simulink model "d_half_bridge_linear_switch_with_basic_diode"  (R2025b)
settings: Solver=VariableStepAuto  StartTime=0.0  StopTime=5/60  RelTol=1e-3
undefined symbols (not defined in the file): DiscIntNeverNeededParam
libraries: fl_lib x8, nesl_utility x4, ee_lib_for_power_systems x2, simulink x1
settings Model: SimulationMode=accelerator  Creator=gdudgeon  LastModifiedBy=gdudgeon

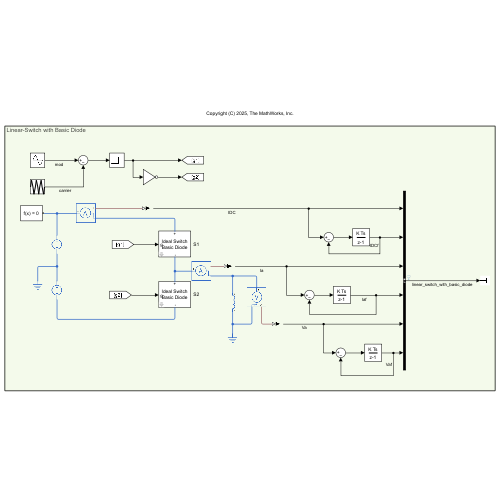
[thumbnail: Simulink's stored preview of the top-level diagram]
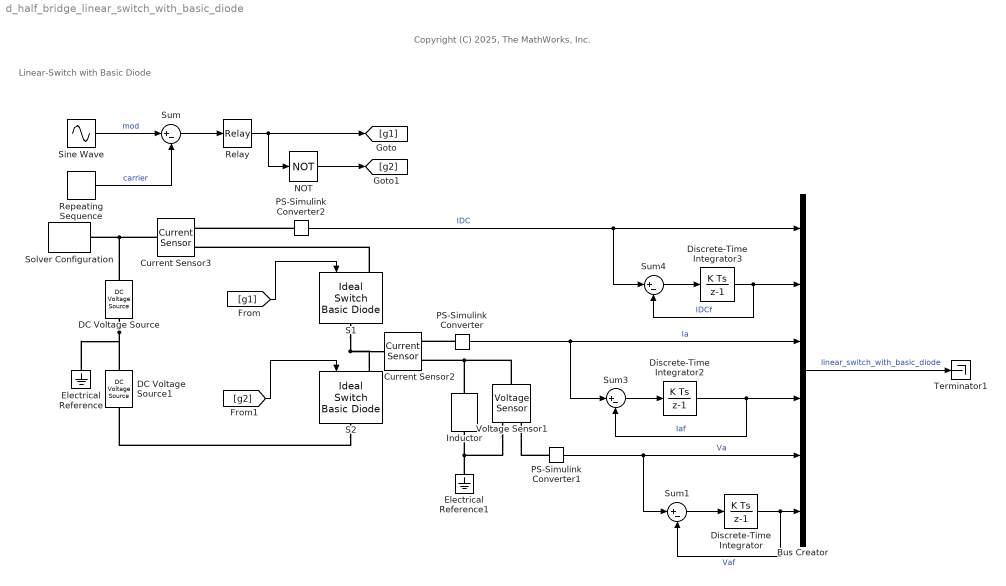
== system d_half_bridge_linear_switch_with_basic_diode ==
  note: Copyright (C) 2025, The MathWorks, Inc.
  note: Linear-Switch with Basic Diode
  Bus Creator : BusCreator  Inputs=6
  Current Sensor2 : fl_lib/Electrical/Electrical Sensors/Current Sensor
  Current Sensor3 : fl_lib/Electrical/Electrical Sensors/Current Sensor
  DC Voltage Source : fl_lib/Electrical/Electrical Sources/DC Voltage Source  v0=50 V
  DC Voltage Source1 : fl_lib/Electrical/Electrical Sources/DC Voltage Source  v0=50 V
  Discrete-Time Integrator : DiscreteIntegrator  gainval=5000  SampleTime=1e-6  ICPrevOutput=DiscIntNeverNeededParam  ICPrevScaledInput=DiscIntNeverNeededParam
  Discrete-Time Integrator2 : DiscreteIntegrator  gainval=5000  SampleTime=1e-6  ICPrevOutput=DiscIntNeverNeededParam  ICPrevScaledInput=DiscIntNeverNeededParam
  Discrete-Time Integrator3 : DiscreteIntegrator  gainval=5000  SampleTime=1e-6  ICPrevOutput=DiscIntNeverNeededParam  ICPrevScaledInput=DiscIntNeverNeededParam
  Electrical Reference : fl_lib/Electrical/Electrical Elements/Electrical Reference
  Electrical Reference1 : fl_lib/Electrical/Electrical Elements/Electrical Reference
  Inductor : fl_lib/Electrical/Electrical Elements/Inductor  l=0.01 H  r=1 Ohm  g=0 1/Ohm  i_specify=off  i_priority=None  i=0 A  i_nominal_specify=off  i_nominal_value=1  i_nominal_unit=A  v_specify=off  v_priority=None  v=0 V  v_nominal_specify=off  v_nominal_value=1  v_nominal_unit=V  i_L_specify=off  i_L_priority=High  i_L=0 A  i_L_nominal_specify=off  i_L_nominal_value=1  i_L_nominal_unit=A
  NOT : Logic  Operator=NOT  IconShape=distinctive  AllPortsSameDT=off  OutDataTypeStr=Inherit: Inherit via back propagation
  PS-Simulink Converter : nesl_utility/PS-Simulink Converter  PhysicalDomain=network_engine_domain  SubClassName=ps_output  LeftPortType=input  RightPortType=output  PseudoPeriodic=off  Frequencies=[]  VectorFormat=inherit  Unit=inherit  AffineConversion=off
  PS-Simulink Converter1 : nesl_utility/PS-Simulink Converter  PhysicalDomain=network_engine_domain  SubClassName=ps_output  LeftPortType=input  RightPortType=output  PseudoPeriodic=off  Frequencies=[]  VectorFormat=inherit  Unit=inherit  AffineConversion=off
  PS-Simulink Converter2 : nesl_utility/PS-Simulink Converter  PhysicalDomain=network_engine_domain  SubClassName=ps_output  LeftPortType=input  RightPortType=output  PseudoPeriodic=off  Frequencies=[]  VectorFormat=inherit  Unit=inherit  AffineConversion=off
  Relay : Relay
  Repeating Sequence : simulink/Sources/Repeating Sequence  rep_seq_t=[0 1 2 3 4]/4/12000  rep_seq_y=[0 1 0 -1 0]
  S1 : ee_lib_for_power_systems/Power Converters/Ideal Switch Basic Diode  Ron=1e-3  Goff=1e-5  run_time=off
      settings: SourceProductName=Support Library for Power Systems
  S2 : ee_lib_for_power_systems/Power Converters/Ideal Switch Basic Diode  Ron=1e-3  Goff=1e-5  run_time=off
      settings: SourceProductName=Support Library for Power Systems
  Sine Wave : Sin  Amplitude=0.8  Frequency=120*pi  SampleTime=0
  Solver Configuration : nesl_utility/Solver Configuration  PhysicalDomain=network_engine_domain  SubClassName=solver  LeftPortType=input  RightPortType=generic  Tones=[]  Harmonics=[]  SimulateNoise=off  Profile=off  UseLocalSampling=off  EnableSwitchedLinearOptims=on  FrequencyDomain=off  UseCCode=off  RelTol=0.001  AbsTol=0.001  MinStep=1e-09  ToWorkspace=off  RevertToSquareIcSolve=off  NumHomotopyIterations=100  PhasorMode=off  PhasorModeNumHarmonics=1  ConsistencySolver=NEWTON_XTOL_AFTER_FTOL  IndexReductionMethod=DerivativeReplacement  DoDC=off  ResidualTolerance=1e-09  ConsistencyTolSource=GLOBAL  ConsistencyAbsTol=0.001  ConsistencyRelTol=0.001  ConsistencyTolFactor=0.001  UseLocalSolver=on  LocalSolverChoice=NE_PARTITIONING_ADVANCER  ResolveIndetEquations=on  FunctionEvalNumThread=1  LocalSolverSampleTime=1e-6  DoFixedCost=off  MaxNonlinIter=3  MaxModeIter=2  ComputeImpulses=off  ImpulseIterations=2  LinearAlgebra=auto  LinearAlgebraNumThread=0  EquationFormulation=NE_TIME_EF  DelaysMemoryBudget=1024  AutomaticFiltering=off  FilteringTimeConstant=0.001  PartitionStorageMethod=AS_NEEDED  PartitionMemoryBudget=1024  PartitionMethod=ROBUST  MultibodyUseLocalSolver=off  MultibodyLocalSolverChoice=ODE1  MultibodyLocalSolverSampleTime=0.001
  Sum{,1,3..4} (4 alike) : Sum  Inputs=|+-
  Terminator1 : Terminator
  Voltage Sensor1 : fl_lib/Electrical/Electrical Sensors/Voltage Sensor
  wires:
  PS-Simulink Converter/1 -> Sum3/1, Bus Creator/3  "Ia"
  Sum1/1 -> Discrete-Time Integrator/1
  Sine Wave/1 -> Sum/1  "mod"
  Sum/1 -> Relay/1
  Discrete-Time Integrator3/1 -> Sum4/2, Bus Creator/2  "IDCf"
  Relay/1 -> NOT/1, [g1]
  Sum3/1 -> Discrete-Time Integrator2/1
  Discrete-Time Integrator/1 -> Bus Creator/6, Sum1/2  "Vaf"
  Repeating Sequence/1 -> Sum/2  "carrier"
  Bus Creator/1 -> Terminator1/1  "linear_switch_with_basic_diode"
  PS-Simulink Converter2/1 -> Sum4/1, Bus Creator/1  "IDC"
  [g2] -> S2/1
  NOT/1 -> [g2]
  Discrete-Time Integrator2/1 -> Bus Creator/4, Sum3/2  "Iaf"
  Sum4/1 -> Discrete-Time Integrator3/1
  PS-Simulink Converter1/1 -> Sum1/1, Bus Creator/5  "Va"
  [g1] -> S1/1
  connections:
  Electrical Reference1/LConn1 -- Voltage Sensor1/RConn2 -- Inductor/RConn1
  S1/RConn1 -- S2/LConn1 -- Current Sensor2/LConn1
  DC Voltage Source/LConn1 -- Current Sensor3/LConn1 -- Solver Configuration/RConn1
  Voltage Sensor1/LConn1 -- Current Sensor2/RConn2 -- Inductor/LConn1
  DC Voltage Source/RConn1 -- DC Voltage Source1/LConn1 -- Electrical Reference/LConn1
  PS-Simulink Converter1/LConn1 -- Voltage Sensor1/RConn1
  PS-Simulink Converter2/LConn1 -- Current Sensor3/RConn1
  PS-Simulink Converter/LConn1 -- Current Sensor2/RConn1
  S1/LConn1 -- Current Sensor3/RConn2
  S2/RConn1 -- DC Voltage Source1/RConn1
